simulink model "bilinear_transformation_high_pass_filter"  (R2020b)
settings: Solver=VariableStepAuto  StartTime=0.0  StopTime=10.0  RelTol=1e-3
settings Model: Creator=user  LastModifiedBy=user

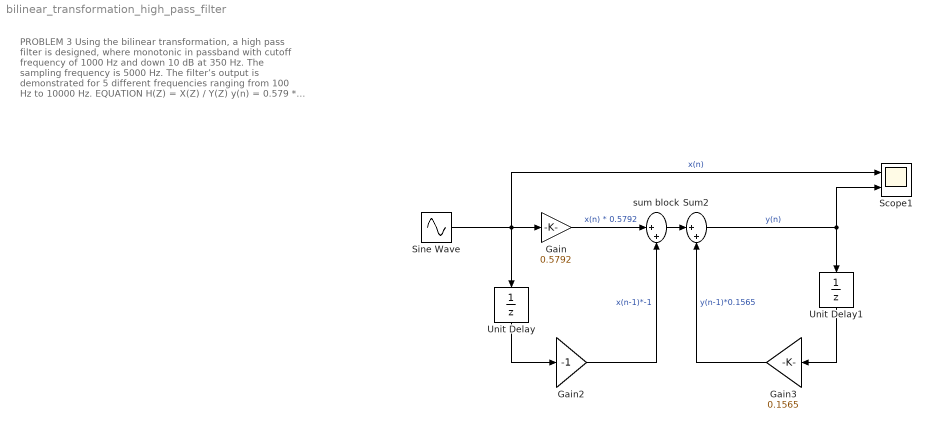
== system bilinear_transformation_high_pass_filter ==
  note: PROBLEM 3
      |
      | Using the bilinear transformation, a high pass filter is designed, where monotonic in passband with cutoff frequency of 1000 Hz and down 10 dB at 350 Hz. The sampling frequency is 5000 Hz. The filter’s output is demonstrated for 5 different frequencies ranging from 100 Hz to 10000 Hz.
      |
      | EQUATION
      | H(Z) = X(Z) / Y(Z)
      | y(n) = 0.579 * x(n)-x(n-1)+0.1565*y(n-1)
  "  Gain2" : Gain  Gain=-1
  " Gain" : Gain  Gain=0.5792
  " Gain3" : Gain  Gain=0.1565
  " Sine Wave" : Sin  Frequency=7000*6.28  SampleTime=0
  " Unit Delay" : UnitDelay  SampleTime=-1  HasFrameUpgradeWarning=on
  " Unit Delay1" : UnitDelay  SampleTime=-1  HasFrameUpgradeWarning=on
  Scope1 : Scope  NumInputPorts=2
  Sum2 : Sum  Inputs=|++
  sum block : Sum  Inputs=|++
  wires:
  " Gain3"/1 -> Sum2/2  "y(n-1)*0.1565"
  " Gain"/1 -> sum block/1  "x(n) * 0.5792"
  " Sine Wave"/1 -> Scope1/1, " Unit Delay"/1, " Gain"/1  "x(n)"
  "  Gain2"/1 -> sum block/2  "x(n-1)*-1"
  " Unit Delay"/1 -> "  Gain2"/1
  " Unit Delay1"/1 -> " Gain3"/1
  Sum2/1 -> Scope1/2, " Unit Delay1"/1  "y(n)"
  sum block/1 -> Sum2/1
